simulink model "Tensegrity_Structure_Small"  (R2022a)
settings: Solver=ode45  StartTime=0.0  StopTime=10  MaxStep=0.001  RelTol=1e-3  AbsTol=1e-3  EnableMultiTasking=on
PreLoadFcn:
  | L=0.3;
  | K=100;
  | D=1;
model workspace (MAT data in the model file):
  L = 1
undefined symbols (not defined in the file or in its folder): X, Y, Z
libraries: sm_lib x243, nesl_utility x43
(part 7 of 7)

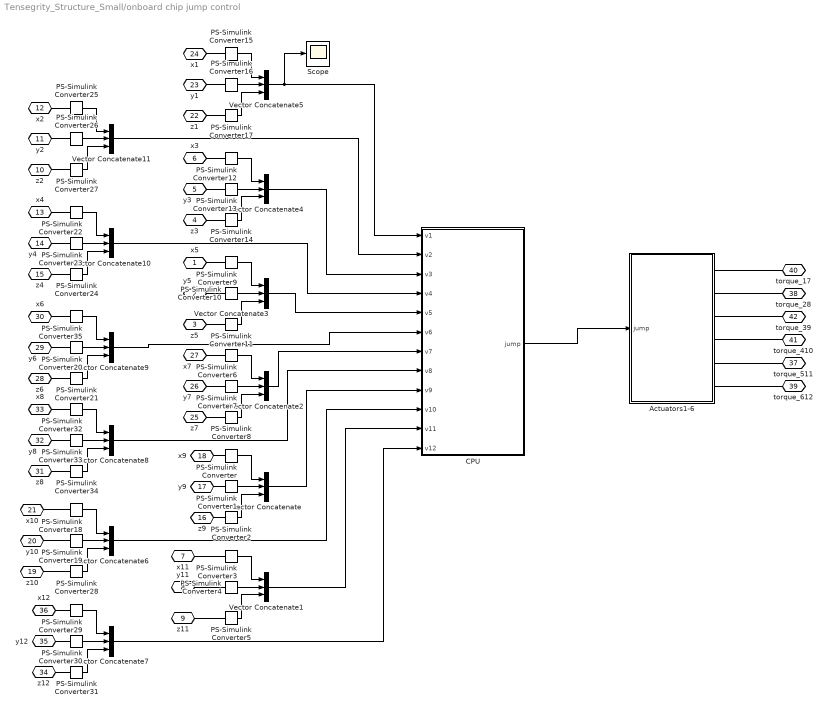
== system Tensegrity_Structure_Small/onboard chip jump control ==
  Actuators1-6 : Subsystem
  CPU : Subsystem
  PS-Simulink Converter{,1..35} (36 alike) : nesl_utility/PS-Simulink Converter  PhysicalDomain=network_engine_domain  SubClassName=ps_output  LeftPortType=input  RightPortType=output  PseudoPeriodic=off  Frequencies=[]  VectorFormat=1-D array  Unit=inherit  AffineConversion=off
      settings: SourceProductBaseCode=SS,PW,VE
  Scope : Scope
  Vector Concatenate{,1..11} (12 alike) : Concatenate  NumInputs=3
  x5 : PMIOPort  Side=Left
  y5 : PMIOPort  Port=2  Side=Left
  z5 : PMIOPort  Port=3  Side=Left
  z3 : PMIOPort  Port=4  Side=Left
  y3 : PMIOPort  Port=5  Side=Left
  x3 : PMIOPort  Port=6  Side=Left
  x11 : PMIOPort  Port=7  Side=Left
  y11 : PMIOPort  Port=8  Side=Left
  z11 : PMIOPort  Port=9  Side=Left
  z2 : PMIOPort  Port=10  Side=Left
  y2 : PMIOPort  Port=11  Side=Left
  x2 : PMIOPort  Port=12  Side=Left
  x4 : PMIOPort  Port=13  Side=Left
  y4 : PMIOPort  Port=14  Side=Left
  z4 : PMIOPort  Port=15  Side=Left
  z9 : PMIOPort  Port=16  Side=Left
  y9 : PMIOPort  Port=17  Side=Left
  x9 : PMIOPort  Port=18  Side=Left
  z10 : PMIOPort  Port=19  Side=Left
  y10 : PMIOPort  Port=20  Side=Left
  x10 : PMIOPort  Port=21  Side=Left
  z1 : PMIOPort  Port=22  Side=Left
  y1 : PMIOPort  Port=23  Side=Left
  x1 : PMIOPort  Port=24  Side=Left
  z7 : PMIOPort  Port=25  Side=Left
  y7 : PMIOPort  Port=26  Side=Left
  x7 : PMIOPort  Port=27  Side=Left
  z6 : PMIOPort  Port=28  Side=Left
  y6 : PMIOPort  Port=29  Side=Left
  x6 : PMIOPort  Port=30  Side=Left
  z8 : PMIOPort  Port=31  Side=Left
  y8 : PMIOPort  Port=32  Side=Left
  x8 : PMIOPort  Port=33  Side=Left
  z12 : PMIOPort  Port=34  Side=Left
  y12 : PMIOPort  Port=35  Side=Left
  x12 : PMIOPort  Port=36  Side=Left
  torque_511 : PMIOPort  Port=37  Side=Right
  torque_28 : PMIOPort  Port=38  Side=Right
  torque_612 : PMIOPort  Port=39  Side=Right
  torque_17 : PMIOPort  Port=40  Side=Right
  torque_410 : PMIOPort  Port=41  Side=Right
  torque_39 : PMIOPort  Port=42  Side=Right
  wires:
  CPU/1(jump) -> Actuators1-6/1(jump)
  PS-Simulink Converter/1 -> Vector Concatenate/1
  PS-Simulink Converter1/1 -> Vector Concatenate/2
  PS-Simulink Converter2/1 -> Vector Concatenate/3
  PS-Simulink Converter5/1 -> Vector Concatenate1/3
  PS-Simulink Converter3/1 -> Vector Concatenate1/1
  PS-Simulink Converter4/1 -> Vector Concatenate1/2
  PS-Simulink Converter8/1 -> Vector Concatenate2/3
  PS-Simulink Converter6/1 -> Vector Concatenate2/1
  PS-Simulink Converter7/1 -> Vector Concatenate2/2
  PS-Simulink Converter11/1 -> Vector Concatenate3/3
  PS-Simulink Converter9/1 -> Vector Concatenate3/1
  PS-Simulink Converter10/1 -> Vector Concatenate3/2
  PS-Simulink Converter14/1 -> Vector Concatenate4/3
  PS-Simulink Converter12/1 -> Vector Concatenate4/1
  PS-Simulink Converter13/1 -> Vector Concatenate4/2
  PS-Simulink Converter17/1 -> Vector Concatenate5/3
  PS-Simulink Converter15/1 -> Vector Concatenate5/1
  PS-Simulink Converter16/1 -> Vector Concatenate5/2
  PS-Simulink Converter30/1 -> Vector Concatenate7/2
  PS-Simulink Converter33/1 -> Vector Concatenate8/2
  PS-Simulink Converter32/1 -> Vector Concatenate8/1
  PS-Simulink Converter34/1 -> Vector Concatenate8/3
  PS-Simulink Converter28/1 -> Vector Concatenate6/3
  PS-Simulink Converter31/1 -> Vector Concatenate7/3
  PS-Simulink Converter27/1 -> Vector Concatenate11/3
  PS-Simulink Converter26/1 -> Vector Concatenate11/2
  PS-Simulink Converter29/1 -> Vector Concatenate7/1
  PS-Simulink Converter35/1 -> Vector Concatenate9/1
  PS-Simulink Converter21/1 -> Vector Concatenate9/3
  PS-Simulink Converter25/1 -> Vector Concatenate11/1
  PS-Simulink Converter20/1 -> Vector Concatenate9/2
  PS-Simulink Converter18/1 -> Vector Concatenate6/1
  PS-Simulink Converter19/1 -> Vector Concatenate6/2
  PS-Simulink Converter24/1 -> Vector Concatenate10/3
  PS-Simulink Converter23/1 -> Vector Concatenate10/2
  PS-Simulink Converter22/1 -> Vector Concatenate10/1
  Vector Concatenate1/1 -> CPU/11(v11)
  Vector Concatenate7/1 -> CPU/12(v12)
  Vector Concatenate/1 -> CPU/9(v9)
  Vector Concatenate6/1 -> CPU/10(v10)
  Vector Concatenate8/1 -> CPU/8(v8)
  Vector Concatenate2/1 -> CPU/7(v7)
  Vector Concatenate9/1 -> CPU/6(v6)
  Vector Concatenate3/1 -> CPU/5(v5)
  Vector Concatenate10/1 -> CPU/4(v4)
  Vector Concatenate4/1 -> CPU/3(v3)
  Vector Concatenate5/1 -> Scope/1, CPU/1(v1)
  Vector Concatenate11/1 -> CPU/2(v2)
  connections:
  Actuators1-6/RConn2 -- torque_28/RConn1
  Actuators1-6/RConn1 -- torque_17/RConn1
  Actuators1-6/RConn6 -- torque_612/RConn1
  Actuators1-6/RConn5 -- torque_511/RConn1
  Actuators1-6/RConn4 -- torque_410/RConn1
  Actuators1-6/RConn3 -- torque_39/RConn1
  z11/RConn1 -- PS-Simulink Converter5/LConn1
  x11/RConn1 -- PS-Simulink Converter3/LConn1
  y11/RConn1 -- PS-Simulink Converter4/LConn1
  z5/RConn1 -- PS-Simulink Converter11/LConn1
  x5/RConn1 -- PS-Simulink Converter9/LConn1
  y5/RConn1 -- PS-Simulink Converter10/LConn1
  z3/RConn1 -- PS-Simulink Converter14/LConn1
  x3/RConn1 -- PS-Simulink Converter12/LConn1
  y3/RConn1 -- PS-Simulink Converter13/LConn1
  z1/RConn1 -- PS-Simulink Converter17/LConn1
  x1/RConn1 -- PS-Simulink Converter15/LConn1
  y1/RConn1 -- PS-Simulink Converter16/LConn1
  x8/RConn1 -- PS-Simulink Converter32/LConn1
  z2/RConn1 -- PS-Simulink Converter27/LConn1
  z12/RConn1 -- PS-Simulink Converter31/LConn1
  y8/RConn1 -- PS-Simulink Converter33/LConn1
  x10/RConn1 -- PS-Simulink Converter18/LConn1
  z8/RConn1 -- PS-Simulink Converter34/LConn1
  x4/RConn1 -- PS-Simulink Converter22/LConn1
  y2/RConn1 -- PS-Simulink Converter26/LConn1
  y10/RConn1 -- PS-Simulink Converter19/LConn1
  x2/RConn1 -- PS-Simulink Converter25/LConn1
  z6/RConn1 -- PS-Simulink Converter21/LConn1
  y12/RConn1 -- PS-Simulink Converter30/LConn1
  z10/RConn1 -- PS-Simulink Converter28/LConn1
  y6/RConn1 -- PS-Simulink Converter20/LConn1
  y4/RConn1 -- PS-Simulink Converter23/LConn1
  z4/RConn1 -- PS-Simulink Converter24/LConn1
  x6/RConn1 -- PS-Simulink Converter35/LConn1
  x12/RConn1 -- PS-Simulink Converter29/LConn1
  PS-Simulink Converter1/LConn1 -- y9/RConn1
  PS-Simulink Converter/LConn1 -- x9/RConn1
  PS-Simulink Converter2/LConn1 -- z9/RConn1
  x7/RConn1 -- PS-Simulink Converter6/LConn1
  y7/RConn1 -- PS-Simulink Converter7/LConn1
  z7/RConn1 -- PS-Simulink Converter8/LConn1

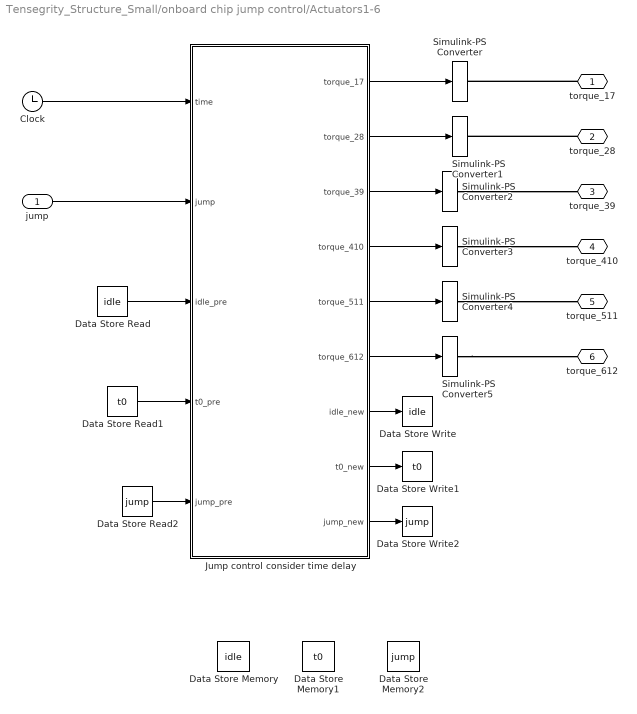
== system Tensegrity_Structure_Small/onboard chip jump control/Actuators1-6 ==
  jump : Inport
  Clock : Clock
  Data Store Memory : DataStoreMemory  DataStoreName=idle  ReadBeforeWriteMsg=warning  WriteAfterWriteMsg=warning  WriteAfterReadMsg=warning  ShowAdditionalParam=off
  Data Store Memory1 : DataStoreMemory  DataStoreName=t0  ReadBeforeWriteMsg=warning  WriteAfterWriteMsg=warning  WriteAfterReadMsg=warning  ShowAdditionalParam=off
  Data Store Memory2 : DataStoreMemory  DataStoreName=jump  ReadBeforeWriteMsg=warning  WriteAfterWriteMsg=warning  WriteAfterReadMsg=warning  InitialValue=[0;0;0;0;0;0]  ShowAdditionalParam=off
  Data Store Read : DataStoreRead  DataStoreName=idle  IndexOptions=Index vector (dialog)  Indices=1  OutputSizes=1
  Data Store Read1 : DataStoreRead  DataStoreName=t0  IndexOptions=Index vector (dialog)  Indices=1  OutputSizes=1
  Data Store Read2 : DataStoreRead  DataStoreName=jump  IndexOptions=Index vector (dialog)  Indices=1  OutputSizes=1
  Data Store Write : DataStoreWrite  DataStoreName=idle  IndexOptions=Index vector (dialog)  Indices=1  OutputSizes=1
  Data Store Write1 : DataStoreWrite  DataStoreName=t0  IndexOptions=Index vector (dialog)  Indices=1  OutputSizes=1
  Data Store Write2 : DataStoreWrite  DataStoreName=jump  IndexOptions=Index vector (dialog)  Indices=1  OutputSizes=1
  Jump control consider time delay : MATLAB Function  TreatAsAtomicUnit=on  SystemSampleTime=0.01
  Simulink-PS Converter{,1..5} (6 alike) : nesl_utility/Simulink-PS Converter  PhysicalDomain=network_engine_domain  SubClassName=ps_input  LeftPortType=input  RightPortType=output  PseudoPeriodic=off  Frequencies=[]  NoiseDistribution=none  NoiseParameters=[]  Unit=1  AffineConversion=off  FilteringAndDerivatives=zero  SimscapeFilterOrder=2  InputFilterTimeConstant=0.001  UdotUserProvided=2
      settings: SourceProductBaseCode=SS,PW,VE
  torque_17 : PMIOPort  Side=Right
  torque_28 : PMIOPort  Port=2  Side=Right
  torque_39 : PMIOPort  Port=3  Side=Right
  torque_410 : PMIOPort  Port=4  Side=Right
  torque_511 : PMIOPort  Port=5  Side=Right
  torque_612 : PMIOPort  Port=6  Side=Right
  wires:
  Jump control consider time delay/1(torque_17) -> Simulink-PS Converter/1
  Clock/1 -> Jump control consider time delay/1(time)
  Jump control consider time delay/2(torque_28) -> Simulink-PS Converter1/1
  jump/1 -> Jump control consider time delay/2(jump)
  Data Store Read/1 -> Jump control consider time delay/3(idle_pre)
  Jump control consider time delay/7(idle_new) -> Data Store Write/1
  Data Store Read1/1 -> Jump control consider time delay/4(t0_pre)
  Jump control consider time delay/8(t0_new) -> Data Store Write1/1
  Jump control consider time delay/9(jump_new) -> Data Store Write2/1
  Data Store Read2/1 -> Jump control consider time delay/5(jump_pre)
  Jump control consider time delay/3(torque_39) -> Simulink-PS Converter2/1
  Jump control consider time delay/4(torque_410) -> Simulink-PS Converter3/1
  Jump control consider time delay/5(torque_511) -> Simulink-PS Converter4/1
  Jump control consider time delay/6(torque_612) -> Simulink-PS Converter5/1
  connections:
  torque_17/RConn1 -- Simulink-PS Converter/RConn1
  torque_28/RConn1 -- Simulink-PS Converter1/RConn1
  Simulink-PS Converter2/RConn1 -- torque_39/RConn1
  Simulink-PS Converter3/RConn1 -- torque_410/RConn1
  Simulink-PS Converter4/RConn1 -- torque_511/RConn1
  Simulink-PS Converter5/RConn1 -- torque_612/RConn1

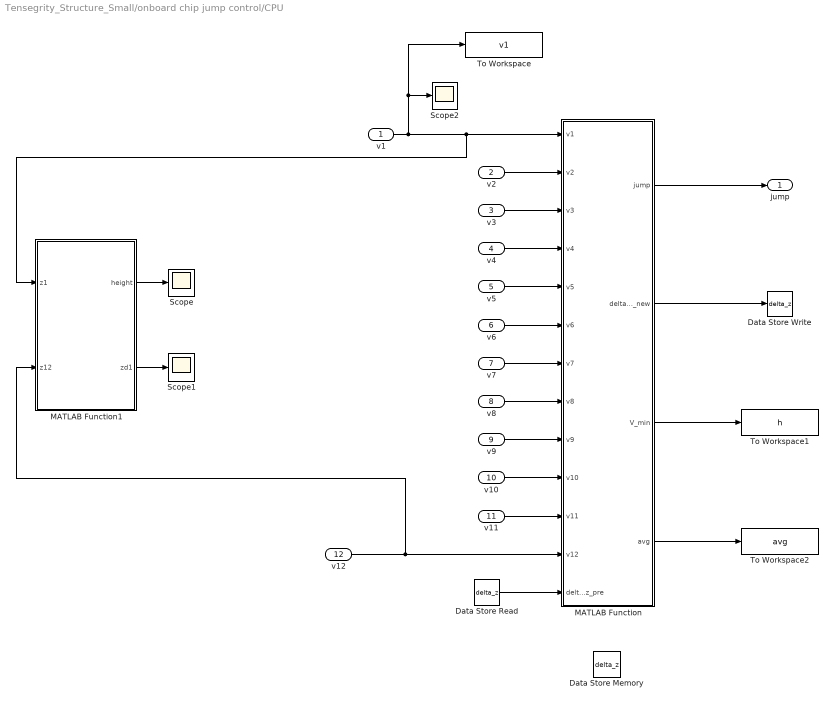
== system Tensegrity_Structure_Small/onboard chip jump control/CPU ==
  v1 : Inport
  v2 : Inport  Port=2
  v3 : Inport  Port=3
  v4 : Inport  Port=4
  v5 : Inport  Port=5
  v6 : Inport  Port=6
  v7 : Inport  Port=7
  v8 : Inport  Port=8
  v9 : Inport  Port=9
  v10 : Inport  Port=10
  v11 : Inport  Port=11
  v12 : Inport  Port=12
  Data Store Memory : DataStoreMemory  DataStoreName=delta_z  ReadBeforeWriteMsg=warning  WriteAfterWriteMsg=warning  WriteAfterReadMsg=warning  InitialValue=[0;0;0;0;0;0]  ShowAdditionalParam=off
  Data Store Read : DataStoreRead  DataStoreName=delta_z  IndexOptions=Index vector (dialog)  Indices=1  OutputSizes=1
  Data Store Write : DataStoreWrite  DataStoreName=delta_z  IndexOptions=Index vector (dialog)  Indices=1  OutputSizes=1
  MATLAB Function : MATLAB Function  TreatAsAtomicUnit=on  SystemSampleTime=0.01
  MATLAB Function1 : MATLAB Function  TreatAsAtomicUnit=on  SystemSampleTime=0.01
  Scope : Scope
  Scope1 : Scope
  Scope2 : Scope
  To Workspace : ToWorkspace  VariableName=v1  SaveFormat=Timeseries  SampleTime=-1
  To Workspace1 : ToWorkspace  VariableName=h  SaveFormat=Timeseries  SampleTime=-1
  To Workspace2 : ToWorkspace  VariableName=avg  SaveFormat=Timeseries  SampleTime=-1
  jump : Outport
  wires:
  MATLAB Function/2(delta_z_new) -> Data Store Write/1
  Data Store Read/1 -> MATLAB Function/13(delta_z_pre)
  v1/1 -> To Workspace/1, Scope2/1, MATLAB Function1/1(z1), MATLAB Function/1(v1)
  MATLAB Function/1(jump) -> jump/1
  MATLAB Function1/1(height) -> Scope/1
  v11/1 -> MATLAB Function/11(v11)
  v12/1 -> MATLAB Function1/2(z12), MATLAB Function/12(v12)
  v2/1 -> MATLAB Function/2(v2)
  v3/1 -> MATLAB Function/3(v3)
  v4/1 -> MATLAB Function/4(v4)
  v5/1 -> MATLAB Function/5(v5)
  v6/1 -> MATLAB Function/6(v6)
  v7/1 -> MATLAB Function/7(v7)
  v8/1 -> MATLAB Function/8(v8)
  v9/1 -> MATLAB Function/9(v9)
  v10/1 -> MATLAB Function/10(v10)
  MATLAB Function1/2(zd1) -> Scope1/1
  MATLAB Function/3(V_min) -> To Workspace1/1
  MATLAB Function/4(avg) -> To Workspace2/1

== matlab function Tensegrity_Structure_Small/onboard chip jump control/Actuators1-6/Jump control consider time delay ==
  data: time input; torque_17 output; jump input; idle_pre input; t0_pre input; torque_28 output; torque_39 output; torque_410 output; torque_511 output; torque_612 output; idle_new output; t0_new output; jump_pre input; jump_new output
function [torque_17,torque_28,torque_39,torque_410,torque_511,torque_612,idle_new,t0_new,jump_new] = jump_delay(time,jump,idle_pre,t0_pre,jump_pre)
%%
t_now = time;
dt = 0.5;
max_torque = 50;
time_delay = 0.00; % discrepancy between 
%%
if idle_pre == 1 % ready to jump
    if max(jump) == 1%jump
        idle_new = 0;
        t0_new = t_now;
        torque_17=0;torque_28=0;torque_39=0;torque_410=0;torque_511=0;torque_612=0;
        jump_new = jump;
    else % no jump
        idle_new = 1;
        t0_new = t_now;
        torque_17=0;torque_28=0;torque_39=0;torque_410=0;torque_511=0;torque_612=0;
        jump_new = zeros(6,1);
    end
   
else % idle_pre == 0;jump in progress
    if t_now <= t0_pre + dt % still have to compress
        idle_new = 0;
        t0_new = t0_pre;
        
        t_in = t_now - t0_pre;
        torque = max_torque*t_in/dt;
        
        torques = torque*jump_pre;  
        torque_17=torques(1);torque_28=torques(2);torque_39=torques(3);torque_410=torques(4);torque_511=torques(5);torque_612=torques(6);
        jump_new = jump_pre;
    elseif t_now <= t0_pre + dt + time_delay % perform delay
        idle_new = 0;
        t0_new = t0_pre;
        
        torque = max_torque;
        
        num_ = find(jump_pre==1,1);% release one bar first
        delay_ = zeros(6,1);
        delay_(num_) = 1;
        jump_delayed = jump_pre - delay_;  
        
        torques = torque*jump_delayed;  
        torque_17=torques(1);torque_28=torques(2);torque_39=torques(3);torque_410=torques(4);torque_511=torques(5);torque_612=torques(6);
        
        jump_new = jump_pre;            
        
    else
        idle_new = 1;
        t0_new = t_now;
        torque_17=0;torque_28=0;torque_39=0;torque_410=0;torque_511=0;torque_612=0;
        jump_new = zeros(6,1);
    end
        
end
    
    
    
    
end % end of function

== matlab function Tensegrity_Structure_Small/onboard chip jump control/CPU/MATLAB Function ==
  data: v1 input; jump output; v2 input; v3 input; v4 input; v5 input; v6 input; v7 input; v8 input; v9 input; v10 input; v11 input; v12 input; delta_z_pre input; delta_z_new output; V_min output; avg output
function [jump, delta_z_new, V_min, avg] = decide(v1,v2,v3,v4,v5,v6,v7,v8,v9,v10,v11,v12,delta_z_pre)
%%
threshold_z = 0.0002;
threshold_dz3 = 25;
isstatic = 0;
%%
dv17 = v1 - v7;
dv28 = v2 - v8;
dv39 = v3 - v9;
dv410 = v4 - v10;
dv511 = v5 - v11;
dv612 = v6 - v12;

% angle1 = 0;
% angle2 = 0;
% angle3 = 0;

% update
v = [dv17 dv28 dv39 dv410 dv511 dv612];
V = [v1(3) v2(3) v3(3) v4(3) v5(3) v6(3) v7(3) v8(3) v9(3) v10(3) v11(3) v12(3)];
plane_pos = [v1(1:2) v2(1:2) v3(1:2) v4(1:2) v5(1:2) v6(1:2) v7(1:2) v8(1:2) v9(1:2) v10(1:2) v11(1:2) v12(1:2)];
avg = [sum(plane_pos(1,:))/12 ; sum(plane_pos(2,:))/12];
V_min = min(V);

delta_z_new = [dv17(3);dv28(3);dv39(3);dv410(3);dv511(3);dv612(3)];
% judge static
n_z = norm(delta_z_new - delta_z_pre);
if n_z < threshold_z % static
    isstatic = 1;
else
    isstatic = 0;
end
% output for mobile/static
if isstatic == 0 %mobile
    jump = zeros(6,1);
else %static
    % determine which two/one bar to jump
    zs = [v1(3);v2(3);v3(3);v4(3);v5(3);v6(3);v7(3);v8(3);v9(3);v10(3);v11(3);v12(3)];
    zs_l2h = sort(zs);% low to high
    min_1 = find(zs==zs_l2h(1)); min_1 = mod(min_1-1,6)+1;
    min_2 = find(zs==zs_l2h(2)); min_2 = mod(min_2-1,6)+1;
    min_3 = find(zs==zs_l2h(3)); min_3 = mod(min_3-1,6)+1; % 1-6
    
    dzs_3 = [abs(delta_z_new(min_1));abs(delta_z_new(min_2));abs(delta_z_new(min_3))];
    
    angle1 = real(acosd(max(min(dot(v(:,min_1),v(:,min_2))/(norm(v(:,min_1))*norm(v(:,min_2))),1),-1)));
    angle2 = real(acosd(max(min(dot(v(:,min_2),v(:,min_3))/(norm(v(:,min_2))*norm(v(:,min_3))),1),-1)));
    angle3 = real(acosd(max(min(dot(v(:,min_3),v(:,min_1))/(norm(v(:,min_3))*norm(v(:,min_1))),1),-1)));

    angles = [angle1 angle2 angle3];
    % sorted = sort(angles);
    if min(angles) < threshold_dz3 % two bars jump
        ids = [min_1;min_2;min_3];
        dontjump_dz = find(dzs_3 == min(dzs_3)); % most horizontal bar doesn't jump
        dontjump_id = ids(dontjump_dz);
        jump = zeros(6,1);
        jump(min_1) = 1;jump(min_2) = 1;jump(min_3) = 1;
        jump(dontjump_id)=0;
      
    else % one bar jump % three bar jump
        jump = zeros(6,1);
        jump(min_1) = 1;
%         jump(min_2) = 1;
%         jump(min_3) = 1;
    end
    delta_z_new = [dv17(3);dv28(3);dv39(3);dv410(3);dv511(3);dv612(3)] + rand(6,1);% in case of static again
end

end %end of function

== matlab function Tensegrity_Structure_Small/onboard chip jump control/CPU/MATLAB Function1 ==
  data: z1 input; height output; z12 input; zd1 output
function [height,zd1]  = cal_height(z1, z12)

height = 0.5*(z1(3)+z12(3));
zd1 = z1(3);
end
